simulink model "Laboratory9"  (R2021b)
settings: Solver=VariableStepAuto  StartTime=0.0  StopTime=10.0  RelTol=1e-3
values from neighbouring files (symbols this model uses):
  Hf1 = tf(2.4,[50.5 1])    [Lab9.m]
  Hf2 = tf(8.6,[0.01*0.6 0.61 1])    [Lab9.m]
  Hr2 = minreal(Ho2/Hf2)    [Lab9.m]
undefined symbols (not defined in the file or in its folder): Hr1f, Hrf
settings Model: Creator=fabian  LastModifiedBy=fabian

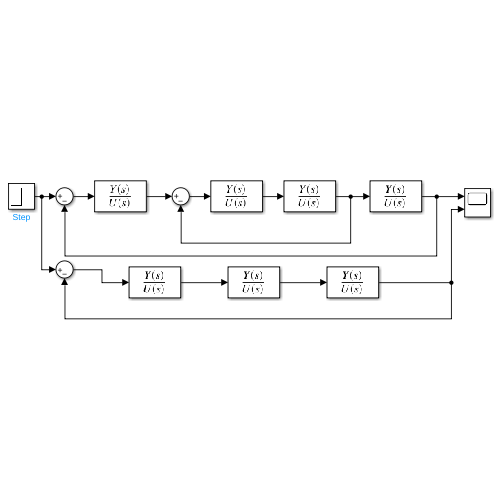
[thumbnail: Simulink's stored preview of the top-level diagram]
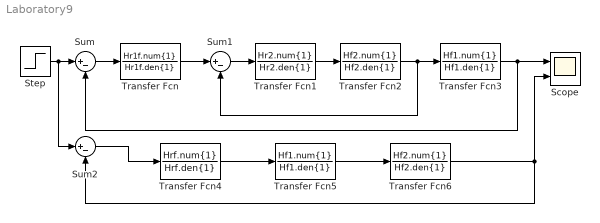
== system Laboratory9 ==
  Scope : Scope  NumInputPorts=2
  Step : Step  SampleTime=0
  Sum : Sum  Inputs=|+-
  Sum1 : Sum  Inputs=|+-
  Sum2 : Sum  Inputs=|+-
  Transfer Fcn : TransferFcn  Numerator=Hr1f.num{1}  Denominator=Hr1f.den{1}
  Transfer Fcn1 : TransferFcn  Numerator=Hr2.num{1}  Denominator=Hr2.den{1}
  Transfer Fcn2 : TransferFcn  Numerator=Hf2.num{1}  Denominator=Hf2.den{1}
  Transfer Fcn3 : TransferFcn  Numerator=Hf1.num{1}  Denominator=Hf1.den{1}
  Transfer Fcn4 : TransferFcn  Numerator=Hrf.num{1}  Denominator=Hrf.den{1}
  Transfer Fcn5 : TransferFcn  Numerator=Hf1.num{1}  Denominator=Hf1.den{1}
  Transfer Fcn6 : TransferFcn  Numerator=Hf2.num{1}  Denominator=Hf2.den{1}
  wires:
  Transfer Fcn2/1 -> Transfer Fcn3/1, Sum1/2
  Transfer Fcn1/1 -> Transfer Fcn2/1
  Sum1/1 -> Transfer Fcn1/1
  Transfer Fcn3/1 -> Sum/2, Scope/1
  Step/1 -> Sum/1, Sum2/1
  Transfer Fcn4/1 -> Transfer Fcn5/1
  Transfer Fcn5/1 -> Transfer Fcn6/1
  Transfer Fcn6/1 -> Sum2/2, Scope/2
  Sum2/1 -> Transfer Fcn4/1
  Sum/1 -> Transfer Fcn/1
  Transfer Fcn/1 -> Sum1/1
